simulink model "chap13_1"  (Simulink 7.9)
settings: Solver=ode45  StartTime=0.0  StopTime=10.0  RelTol=1e-3
libraries: simulink x5
settings Model: Creator=lenovo  LastModifiedBy=lenovo

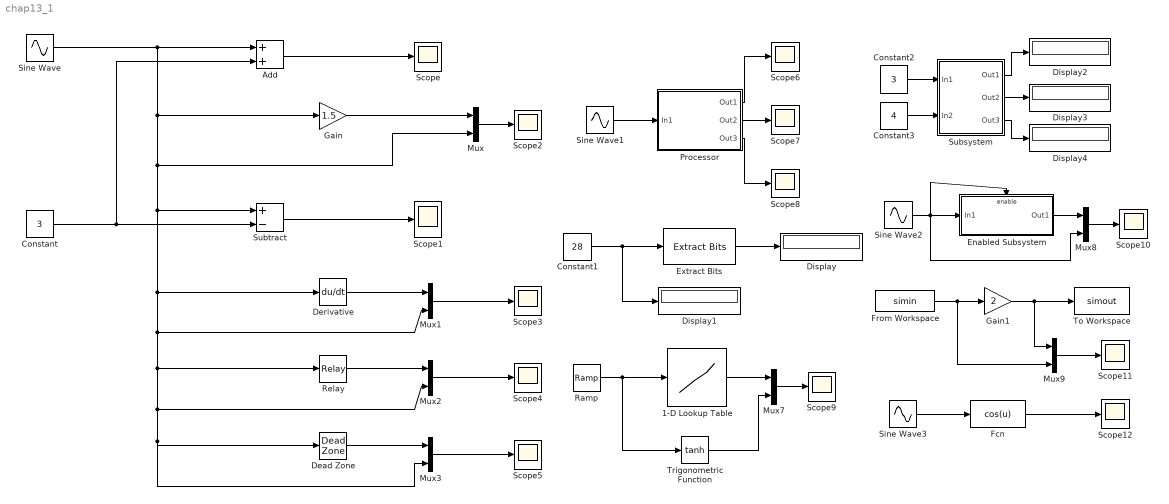
== system chap13_1 ==
  1-D Lookup Table : Lookup_n-D  NumberOfTableDimensions=1  BreakpointsForDimension1=[-5:5]  Table=tanh([-5:5])  RndMeth=Simplest  InputSameDT=on
  Add : Sum
  Constant : Constant  Value=3
  Constant1 : Constant  Value=28  OutDataTypeStr=int8
  Constant2 : Constant  Value=3  OutDataTypeStr=double
  Constant3 : Constant  Value=4  OutDataTypeStr=double
  Dead Zone : DeadZone  SaturateOnIntegerOverflow=on
  Derivative : Derivative
  Display{,1..4} (5 alike) : Display
      Display settings: Format=binary (Stored Integer)
      Display1 settings: Format=binary (Stored Integer)
  Enabled Subsystem : Subsystem  TreatAsAtomicUnit=on
  Extract Bits : simulink/Logic and Bit Operations/Extract Bits  bitsToExtract=Upper half  numBits=8  bitIdxRange=[0 7]  outScalingMode=Preserve fixed-point scaling
  Fcn : Fcn  Expr=cos(u)
  From Workspace : FromWorkspace  VariableName=simin  SampleTime=0
  Gain : Gain  Gain=1.5
  Gain1 : Gain  Gain=2
  Mux{,1..3,7..9} (7 alike) : Mux  Inputs=2
      Mux9 settings: DisplayOption=signals
  Processor : Subsystem  mask(complex processor for signal){m=3}
      mask prompts: m "Gain Value"
      mask help: A simplify example for simulink!
      mask Display:
      | port_label('input',1,'single');
      | port_label('output',1,'Diff');
      | port_label('output',2,'Disc');
      | port_label('output',3,'Data');
      | image(imread('b747.jpg'))
  Ramp : simulink/Sources/Ramp  slope=2  start=-5  X0=5
  Relay : Relay
  Scope{,1..12} (13 alike) : Scope
      Scope10 settings: TimeRange=10  YMin=-1  YMax=2  SaveName=ScopeData10
      Scope11 settings: TimeRange=10  YMin=0.999  YMax=1.009  SaveName=ScopeData11
      Scope12 settings: TimeRange=10  YMin=0.999  YMax=1.009  SaveName=ScopeData12
      Scope2 settings: SaveName=ScopeData2
      Scope3 settings: SaveName=ScopeData3
      Scope4 settings: SaveName=ScopeData4
      Scope5 settings: SaveName=ScopeData5
      Scope6 settings: SaveName=ScopeData6
      Scope7 settings: SaveName=ScopeData7
      Scope8 settings: SaveName=ScopeData8
      Scope9 settings: TimeRange=10  YMin=0.999  YMax=1.009  SaveName=ScopeData9
  Sine Wave : Sin  SampleTime=0.01
  Sine Wave1 : Sin  SampleTime=0.2
  Sine Wave2 : Sin  SampleTime=0.01
  Sine Wave3 : Sin  SampleTime=0.01
  Subsystem : Subsystem
      mask Type: A complex number transform to real an image
      mask Description: usefull to transform to real an image
      mask Display:
      | port_label('input',1,'real');
      | port_label('input',2,'imag');
      | port_label('output',1,'abs');
      | port_label('output',2,'angel');
      | port_label('output',3,'complex');
  Subtract : Sum  Inputs=+-
  To Workspace : ToWorkspace  VariableName=simout  SampleTime=-1
  Trigonometric Function : Trigonometry  Operator=tanh
  wires:
  Sine Wave/1 -> Add/1, Gain/1, Mux/2, Subtract/1, Derivative/1, Mux1/2, Relay/1, Mux2/2, Dead Zone/1, Mux3/2
  Constant/1 -> Subtract/2, Add/2
  Add/1 -> Scope/1
  Subtract/1 -> Scope1/1
  Gain/1 -> Mux/1
  Mux/1 -> Scope2/1
  Mux1/1 -> Scope3/1
  Derivative/1 -> Mux1/1
  Mux3/1 -> Scope5/1
  Mux2/1 -> Scope4/1
  Relay/1 -> Mux2/1
  Dead Zone/1 -> Mux3/1
  Processor/1(Out1) -> Scope6/1
  Processor/2(Out2) -> Scope7/1
  Processor/3(Out3) -> Scope8/1
  Extract Bits/1 -> Display/1
  Constant1/1 -> Extract Bits/1, Display1/1
  Ramp/1 -> 1-D Lookup Table/1, Trigonometric Function/1
  1-D Lookup Table/1 -> Mux7/1
  Trigonometric Function/1 -> Mux7/2
  Mux7/1 -> Scope9/1
  Constant2/1 -> Subsystem/1(In1)
  Constant3/1 -> Subsystem/2(In2)
  Sine Wave2/1 -> Enabled Subsystem/1(In1), Mux8/2, Enabled Subsystem/Enable
  Mux8/1 -> Scope10/1
  Enabled Subsystem/1(Out1) -> Mux8/1
  Mux9/1 -> Scope11/1
  Gain1/1 -> To Workspace/1, Mux9/1
  From Workspace/1 -> Gain1/1, Mux9/2
  Sine Wave1/1 -> Processor/1(In1)
  Subsystem/3(Out3) -> Display4/1
  Subsystem/2(Out2) -> Display3/1
  Subsystem/1(Out1) -> Display2/1
  Sine Wave3/1 -> Fcn/1
  Fcn/1 -> Scope12/1

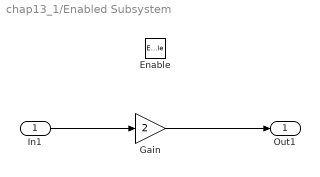
== system chap13_1/Enabled Subsystem ==
  In1 : Inport
  Enable : EnablePort
  Gain : Gain  Gain=2
  Out1 : Outport
  wires:
  In1/1 -> Gain/1
  Gain/1 -> Out1/1

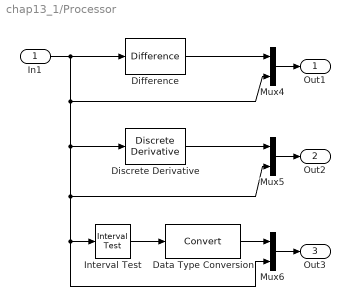
== system chap13_1/Processor ==
  In1 : Inport
  Data Type Conversion : DataTypeConversion
  Difference : simulink/Discrete/Difference  ICPrevInput=0.0  InputProcessing=Inherited  OutMin=[]  OutMax=[]  OutDataType=fixdt(1, 16)  OutScaling=2^-10  DoSatur=off
  Discrete Derivative : simulink/Discrete/Discrete Derivative  gainval=2.0  ICPrevScaledInput=0.0  InputProcessing=Inherited  OutMin=[]  OutMax=[]  OutDataType=fixdt(1, 16)  OutScaling=2^-10  DoSatur=off
  Interval Test : simulink/Logic and Bit Operations/Interval Test  IntervalClosedRight=on  uplimit=0.5  IntervalClosedLeft=on  lowlimit=-0.5  OutDataTypeStr=boolean
  Mux4 : Mux  Inputs=2
  Mux5 : Mux  Inputs=2
  Mux6 : Mux  Inputs=2
  Out1 : Outport
  Out2 : Outport  Port=2
  Out3 : Outport  Port=3
  wires:
  Data Type Conversion/1 -> Mux6/1
  Discrete Derivative/1 -> Mux5/1
  Difference/1 -> Mux4/1
  In1/1 -> Difference/1, Discrete Derivative/1, Interval Test/1, Mux6/2, Mux5/2, Mux4/2
  Interval Test/1 -> Data Type Conversion/1
  Mux4/1 -> Out1/1
  Mux5/1 -> Out2/1
  Mux6/1 -> Out3/1

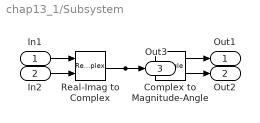
== system chap13_1/Subsystem ==
  In1 : Inport
  In2 : Inport  Port=2
  Complex to Magnitude-Angle : ComplexToMagnitudeAngle
  Real-Imag to Complex : RealImagToComplex
  Out1 : Outport
  Out2 : Outport  Port=2
  Out3 : Outport  Port=3
  wires:
  Real-Imag to Complex/1 -> Complex to Magnitude-Angle/1, Out3/1
  Complex to Magnitude-Angle/1 -> Out1/1
  In1/1 -> Real-Imag to Complex/1
  Complex to Magnitude-Angle/2 -> Out2/1
  In2/1 -> Real-Imag to Complex/2
